simulink model "DataCenterCooling"  (R2025b)
settings: Solver=daessc  StartTime=0.0  StopTime=(env.nDays-1)*24*3600  MaxStep=60  RelTol=1e-3  AbsTol=1e-3
PreLoadFcn:
  | run("DataCenterCoolingExampleParams")
undefined symbols (not defined in the file or in its folder): cdu, Datacenter, ModelDatacenterLiquidCooling
libraries: fl_lib x101, SimscapeFluids_lib x27, nesl_utility x21, datacenter_lib x13, simulink_extras x2, slpidlib x1, buildingEnergy_lib x1
(part 1 of 3)
CloseFcn:
  | clear tout env cdu
Description:
  | Data Center Cooling
settings Model: Creator=The MathWorks, Inc.  LastModifiedBy=skota
settings SolverCC: AutoScaleAbsTol=off  MaxConsecutiveMinStep=500  AlgebraicLoopSolver=TrustRegion  MaxZcPerStep=1.0
settings DataIOCC: SaveOutput=off  DSMLogging=off  SaveTime=off  ReturnWorkspaceOutputs=off  SignalLoggingName=measurement_DataCenterCooling
settings OptimizationCC: ReuseModelBlockBuffer=off
settings DebuggingCC: UnconnectedInputMsg=warning  UnconnectedOutputMsg=warning  UnconnectedLineMsg=warning  SymbolicDimsDataTypeCodeGenerationDiagnostic=none
settings ModelReferenceCC: EnableRefExpFcnMdlSchedulingChecks=on
settings SFSimCC: CustomCodeUndefinedFunction=UseInterfaceOnly
settings RTWCC: GPUComputeCapability=3.5  DLArmComputeVersion=19.05
settings SimscapeCC: SimscapeLogType=all  SimscapeLogSimulationStatistics=on  SimscapeLogName=simlog_DataCenterCooling  SimscapeLogDataHistory=50000.0  SimscapeCompileComponentReuse=on

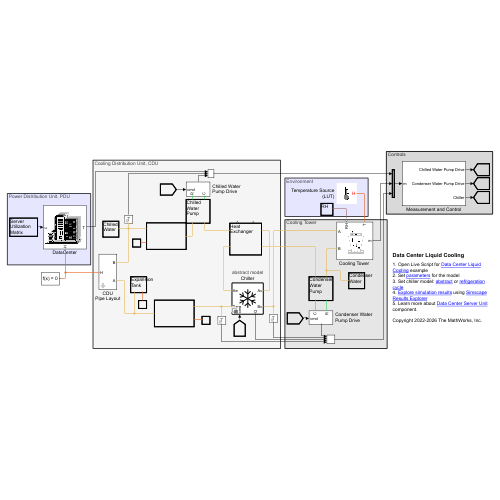
[thumbnail: Simulink's stored preview of the top-level diagram]
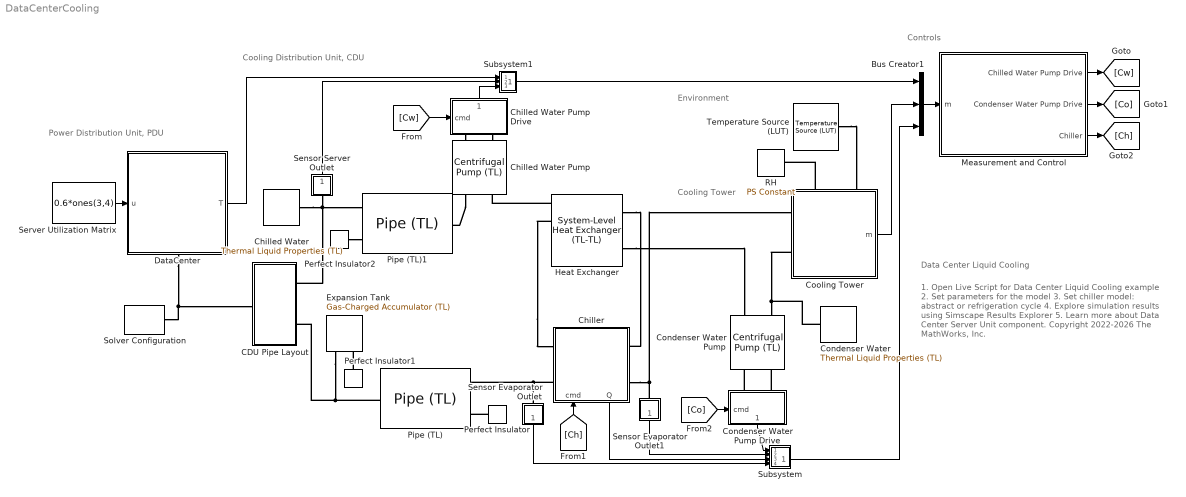
== system DataCenterCooling ==
  note: Controls
  note: Cooling Tower
  note: Environment
  note: Power Distribution Unit, PDU
  note: Cooling Distribution Unit, CDU
  note: Data Center Liquid Cooling
  note: 1. Open Live Script for Data Center Liquid Cooling example
      | 2. Set parameters for the model
      | 3. Set chiller model: abstract or refrigeration cycle
      | 4. Explore simulation results using Simscape Results Explorer
      | 5. Learn more about Data Center Server Unit component.
      |
      | Copyright 2022-2026 The MathWorks, Inc.
  Bus Creator1 : BusCreator  Inputs=3
  CDU Pipe Layout : Subsystem  mask{thRes=1e-5, distrDiameter=0.2, pipeDiameter=0.05, pipeLength=5}
      mask prompts: thRes "Thermal resistance (K/W)"; distrDiameter "Distributor pipe diameter (m)"; pipeDiameter "Cooling pipe diameter"; pipeLength "Pipe length (m)"
  Chilled Water : SimscapeFluids_lib/Thermal Liquid/Utilities/Thermal Liquid Properties (TL)  fluid_list=fluids.thermal_liquid.utilities.enum.thermal_liquid_fluid_list.ethylene_glycol  concentration_param_EG=fluids.thermal_liquid.utilities.enum.thermal_liquid_concentration.volume_fraction  concentration_param_PG=fluids.thermal_liquid.utilities.enum.thermal_liquid_concentration.volume_fraction  c_mass_SW=3.5e-3  c_mass_EG=0.1  c_mass_PG=0.1  c_mass_GL=0.1  c_vol_EG=0.3  c_vol_PG=0.1  beta_const_EG=2.1791 GPa  beta_const_PG=2.1791 GPa  beta_const_GL=2.1791 GPa  p_min_EG=0.01 MPa  p_min_PG=0.01 MPa  p_min_GL=0.01 MPa  p_max_EG=50 MPa  p_max_PG=50 MPa  p_max_GL=50 MPa  T_atm=293.15 K  p_atm=0.101325 MPa  properties_range_check=simscape.enum.assert.action.error  air_fraction=0  R_air=0.287 kJ/(K*kg)  air_dissolution_model=false  p_crit=3 MPa
  Chilled Water Pump : SimscapeFluids_lib/Thermal Liquid/Pumps & Motors/Centrifugal Pump (TL)  pump_parameterization=fluids.thermal_liquid.pumps_motors.enum.CentrifugalPumpParameterization.Nominal  capacity_ref_nominal=9600 lpm  head_ref_nominal=28 m  power_ref_nominal=60 kW  head_ref_max=40 m  capacity_ref_max=15000 lpm  omega_ref_analytic=2400 rpm  flow_rate_1D_TLU=[16.67, 30, 40, 53.33, 66.67, 83.33] lpm  head_1D_TLU=[50, 47.5, 45, 40, 35, 25] m  power_1D_TLU=[.6, .75, .85, .93, .98, .99] kW  omega_ref_1D=3500 rpm  rho_ref_1D=998.21 kg/m^3  omega_threshold_factor=1e-2  flow_rate_2D_TLU=[16.67, 23.33, 30, 40, 53.33, 60] lpm  omega_2D_TLU=[2450, 2800, 3150, 3500] rpm  head_2D_TLU=[25, 32.7, 42.5, 50; 24, 31.7, 41, 49; 22.7, 30.5, 39, 47.5; 20, 28, 36, 45; 15.7, 24, 32, 40; 12.5, 21, 29.5, 37.5] m  power_2D_TLU=[.28, .38, .5, .6; .31, .41, .55, .68; .33, .44, .6, .75; .36, .48, .65, .83; .38, .53, .72, .93; .39, .55, .75, .97] kW  rho_ref_2D=998.21 kg/m^3  diameter_ratio=1  mech_orientation=fluids.thermal_liquid.pumps_motors.enum.CentrifugalPumpMechOrientation.Positive  area=cdu.port_area m^2  operation_check=simscape.enum.assert.action.none
  Chilled Water Pump Drive : Subsystem
      settings: PortSchema="{\"entries\":[{\"content\":{\"sides\":[{\"content\":{},\"type\":\"ConnectorPlacement.EquallySpacedRectSide\",\"uuid\":\"edaea338-c02b-45e4-bb82-2d3d355c0ecb\"},{\"content\":{\"connectorIds\":[\"In1\"],\"side\":\"RIGHT\"},\"type\":\"ConnectorPlacement.EquallySpacedRectSide\",\"uuid\":\"dbf9c5c1-eafd-40d4-aa46-26e8ea9aa192\"},{\"content\":{\"connectorIds\":[\"LConn1\",\"LConn2\"],\"side\":\"TOP\"},\"type\":\"ConnectorPlacement.EquallySpacedRectSide\",\"uuid\":\"608efdba-9ff5-4da4-84d8-d12421fbb1b5\"},{\"content\":{\"connectorIds\":[\"Out1\"],\"side\":\"BOTTOM\"},\"type\":\"ConnectorPlacement.EquallySpacedRectSide\",\"uuid\":\"72b6a2af-375d-4ab8-a644-645304dfa2ef\"}]},\"type\":\"ConnectorPlacement.EquallySpacedConnector\",\"uuid\":\"d68ea5d9-0a41-4434-9ea5-6f17886b9eb3\"}],\"packageUris\":[\"http://schema.mathworks.com/mf0/Connector/R2020b\"],\"version\":\"1.0\"}"
  Chiller : Subsystem  Variant=on  VariantControlMode=label  LabelModeActiveChoice=abstract model
      settings: AttributesFormatString=%<LabelModeActiveChoice>  PortSchema="{\"entries\":[{\"content\":{\"sides\":[{\"content\":{\"connectorIds\":[\"LConn1\",\"LConn2\"]},\"type\":\"ConnectorPlacement.EquallySpacedRectSide\",\"uuid\":\"5ef38cea-bb7b-401a-87d4-4f5e5e2c1e9f\"},{\"content\":{\"connectorIds\":[\"RConn1\",\"RConn2\"],\"side\":\"RIGHT\"},\"type\":\"ConnectorPlacement.EquallySpacedRectSide\",\"uuid\":\"7c200196-8d5a-4dde-899e-2352968f9ffc\"},{\"content\":{\"side\":\"TOP\"},\"type\":\"ConnectorPlacement.EquallySpacedRectSide\",\"uuid\":\"5e8cb91d-7f29-4d1c-a98e-548e0eb69733\"},{\"content\":{\"connectorIds\":[\"In1\",\"Out1\"],\"side\":\"BOTTOM\"},\"type\":\"ConnectorPlacement.EquallySpacedRectSide\",\"uuid\":\"d3cfe7a1-f14c-45f3-9f19-8fd891085d29\"}]},\"type\":\"ConnectorPlacement.EquallySpacedConnector\",\"uuid\":\"25b6c22e-1b50-48b1-b598-85423fadd037\"}],\"packageUris\":[\"http://schema.mathworks.com/mf0/Connector/R2020b\"],\"version\":\"1.0\"}"
      mask Display:
      | plot([-100 100 100 -100 -100], [-100 -100 100 100 -100])
      | 
      | % Width and height scale factors
      | w = 60;
      | h = 60;
      | 
      | % Coordinates [x; y]
      | trunk = [0 0; -1 1];
      | tip1 = [-0.3 0 0.3; 0.8 0.5 0.8];
      | tip2 = [-0.3 0 0.3; -0.8 -0.5 -0.8];
      | 
      | % Vertical line
      | plot(w*trunk(1,:), h*trunk(2,:))
      | plot(w*tip1(1,:), h*tip1(2,:))
      | plot(w*tip2(1,:), h*tip2(2,:))
      | 
      | % Rotate 60 deg
      | theta = 60;
      | rot = [cosd(theta) -sind(theta); sind(theta) cosd(theta)];
      | trunk_rot = rot*trunk;
      | tip1_rot = rot*tip1;
      | tip2_rot = rot*tip2;
      | plot(w*trunk_rot(1,:), h*trunk_rot(2,:))
      | plot(w*tip1_rot(1,:), h*tip1_rot(2,:))
      | plot(w*tip2_rot(1,:), h*tip2_rot(2,:))
      | 
      | % Rotate 120 deg
      | theta = 120;
      | rot = [cosd(theta) -sind(theta); sind(theta) cosd(theta)];
      | trunk_rot = rot*trunk;
      | tip1_rot = rot*tip1;
      | tip2_rot = rot*tip2;
      | plot(w*trunk_rot(1,:), h*trunk_rot(2,:))
      | plot(w*tip1_rot(1,:), h*tip1_rot(2,:))
      | plot(w*tip2_rot(1,:), h*tip2_rot(2,:))
  Condenser Water : SimscapeFluids_lib/Thermal Liquid/Utilities/Thermal Liquid Properties (TL)  fluid_list=fluids.thermal_liquid.utilities.enum.thermal_liquid_fluid_list.water  concentration_param_EG=fluids.thermal_liquid.utilities.enum.thermal_liquid_concentration.volume_fraction  concentration_param_PG=fluids.thermal_liquid.utilities.enum.thermal_liquid_concentration.volume_fraction  c_mass_SW=3.5e-3  c_mass_EG=0.1  c_mass_PG=0.1  c_mass_GL=0.1  c_vol_EG=0.1  c_vol_PG=0.1  beta_const_EG=2.1791 GPa  beta_const_PG=2.1791 GPa  beta_const_GL=2.1791 GPa  p_min_EG=0.01 MPa  p_min_PG=0.01 MPa  p_min_GL=0.01 MPa  p_max_EG=50 MPa  p_max_PG=50 MPa  p_max_GL=50 MPa  T_atm=293.15 K  p_atm=0.101325 MPa  properties_range_check=simscape.enum.assert.action.error  air_fraction=0  R_air=0.287 kJ/(K*kg)  air_dissolution_model=false  p_crit=3 MPa
  Condenser Water Pump : SimscapeFluids_lib/Thermal Liquid/Pumps & Motors/Centrifugal Pump (TL)  pump_parameterization=fluids.thermal_liquid.pumps_motors.enum.CentrifugalPumpParameterization.Nominal  capacity_ref_nominal=15000 lpm  head_ref_nominal=33 m  power_ref_nominal=100 kW  head_ref_max=48 m  capacity_ref_max=24000 lpm  omega_ref_analytic=2400 rpm  flow_rate_1D_TLU=[16.67, 30, 40, 53.33, 66.67, 83.33] lpm  head_1D_TLU=[50, 47.5, 45, 40, 35, 25] m  power_1D_TLU=[.6, .75, .85, .93, .98, .99] kW  omega_ref_1D=3500 rpm  rho_ref_1D=998.21 kg/m^3  omega_threshold_factor=1e-2  flow_rate_2D_TLU=[16.67, 23.33, 30, 40, 53.33, 60] lpm  omega_2D_TLU=[2450, 2800, 3150, 3500] rpm  head_2D_TLU=[25, 32.7, 42.5, 50; 24, 31.7, 41, 49; 22.7, 30.5, 39, 47.5; 20, 28, 36, 45; 15.7, 24, 32, 40; 12.5, 21, 29.5, 37.5] m  power_2D_TLU=[.28, .38, .5, .6; .31, .41, .55, .68; .33, .44, .6, .75; .36, .48, .65, .83; .38, .53, .72, .93; .39, .55, .75, .97] kW  rho_ref_2D=998.21 kg/m^3  diameter_ratio=1  mech_orientation=fluids.thermal_liquid.pumps_motors.enum.CentrifugalPumpMechOrientation.Positive  area=cdu.port_area m^2  operation_check=simscape.enum.assert.action.none
  Condenser Water Pump Drive : Subsystem
      settings: PortSchema="{\"entries\":[{\"content\":{\"sides\":[{\"content\":{\"connectorIds\":[\"In1\"]},\"type\":\"ConnectorPlacement.EquallySpacedRectSide\",\"uuid\":\"edaea338-c02b-45e4-bb82-2d3d355c0ecb\"},{\"content\":{\"side\":\"RIGHT\"},\"type\":\"ConnectorPlacement.EquallySpacedRectSide\",\"uuid\":\"dbf9c5c1-eafd-40d4-aa46-26e8ea9aa192\"},{\"content\":{\"connectorIds\":[\"LConn1\",\"LConn2\"],\"side\":\"TOP\"},\"type\":\"ConnectorPlacement.EquallySpacedRectSide\",\"uuid\":\"608efdba-9ff5-4da4-84d8-d12421fbb1b5\"},{\"content\":{\"connectorIds\":[\"Out1\"],\"side\":\"BOTTOM\"},\"type\":\"ConnectorPlacement.EquallySpacedRectSide\",\"uuid\":\"608ab80a-f5e8-4836-b78e-f2f30ba8946b\"}]},\"type\":\"ConnectorPlacement.EquallySpacedConnector\",\"uuid\":\"d68ea5d9-0a41-4434-9ea5-6f17886b9eb3\"}],\"packageUris\":[\"http://schema.mathworks.com/mf0/Connector/R2020b\"],\"version\":\"1.0\"}"
  "Cooling Tower " : Subsystem
      settings: PortSchema="{\"entries\":[{\"content\":{\"sides\":[{\"content\":{\"connectorIds\":[\"LConn1\",\"LConn2\"]},\"type\":\"ConnectorPlacement.EquallySpacedRectSide\",\"uuid\":\"fb95f023-248b-4fd8-b2e8-d9442f9ed266\"},{\"content\":{\"connectorIds\":[\"Out1\"],\"side\":\"RIGHT\"},\"type\":\"ConnectorPlacement.EquallySpacedRectSide\",\"uuid\":\"34018b48-7083-4d8d-9b59-330dd3458507\"},{\"content\":{\"connectorIds\":[\"LConn3\",\"LConn4\"],\"side\":\"TOP\"},\"type\":\"ConnectorPlacement.EquallySpacedRectSide\",\"uuid\":\"5b7035e5-549d-4a54-bb0d-bc476d1d6775\"}]},\"type\":\"ConnectorPlacement.EquallySpacedConnector\",\"uuid\":\"c33b1996-e402-4893-a457-f5cd841aa14c\"}],\"packageUris\":[\"http://schema.mathworks.com/mf0/Connector/R2020b\"],\"version\":\"1.0\"}"
      mask Display: image('coolingTowerIcon.png');
  DataCenter : Subsystem
      settings: PortSchema="{\"entries\":[{\"content\":{\"sides\":[{\"content\":{\"connectorIds\":[\"In1\"]},\"type\":\"ConnectorPlacement.EquallySpacedRectSide\",\"uuid\":\"0d94ea3d-d897-456d-b7bd-42d620e46e28\"},{\"content\":{\"connectorIds\":[\"Out1\"],\"side\":\"RIGHT\"},\"type\":\"ConnectorPlacement.EquallySpacedRectSide\",\"uuid\":\"b45d02ac-efb1-4fbd-bb62-56ba599fe73d\"},{\"content\":{\"side\":\"TOP\"},\"type\":\"ConnectorPlacement.EquallySpacedRectSide\",\"uuid\":\"5c5ba700-ead5-48ef-be98-ffdeec5238e7\"},{\"content\":{\"connectorIds\":[\"RConn1\"],\"side\":\"BOTTOM\"},\"type\":\"ConnectorPlacement.EquallySpacedRectSide\",\"uuid\":\"4fcdfdd2-a15c-4a40-81f5-7d3c5a9fd94e\"}]},\"type\":\"ConnectorPlacement.EquallySpacedConnector\",\"uuid\":\"41bff309-caa4-4da4-abd9-c4b3acd5f02a\"}],\"packageUris\":[\"http://schema.mathworks.com/mf0/Connector/R2020b\"],\"version\":\"1.0\"}"
      mask Display: image('datacenter.png');
  Expansion Tank : SimscapeFluids_lib/Thermal Liquid/Tanks & Accumulators/Gas-Charged Accumulator (TL)  capacity=1 m^3  dead_volume=1e-3 m^3  p_precharge_gauge=0.28 MPa  k_sh=1.4  area=cdu.port_area m^2  stiff_coeff=1e4 MPa/m^3  damping_coeff=1e4 MPa*s/m^6  liquid_volume_specify=on  liquid_volume_priority=None  liquid_volume=5e-3 m^3  liquid_volume_nominal_specify=off  liquid_volume_nominal_value=1  liquid_volume_nominal_unit=m^3  liquid_mass_specify=off  liquid_mass_priority=None  liquid_mass=5 kg  liquid_mass_nominal_specify=off  liquid_mass_nominal_value=1  liquid_mass_nominal_unit=kg  p_I_specify=on  p_I_priority=High  p_I=0.4 MPa  p_I_nominal_specify=off  p_I_nominal_value=1  p_I_nominal_unit=MPa  T_I_specify=on  T_I_priority=High  T_I=18 degC  T_I_nominal_specify=off  T_I_nominal_value=1  T_I_nominal_unit=K
  Heat Exchanger : SimscapeFluids_lib/Heat Exchangers/Thermal Liquid/System-Level Heat Exchanger (TL-TL)  flow_arrangement=fluids.heat_exchangers.enum.SystemLevelFlowArrangementTLTL.Counter  wall_thermal_mass=false  mass_wall=1 kg  cp_wall=490 J/(K*kg)  nominal_init_wall=true  T_wall_init=293.15 K  area_A1=cdu.port_area m^2  area_B1=cdu.port_area m^2  area_A2=cdu.port_area m^2  area_B2=cdu.port_area m^2  operating_condition_TL1=fluids.heat_exchangers.enum.SystemLevelOperatingConditionTLTL.Cooling  mdot_nominal_TL1=160 kg/s  delta_p_nominal_TL1=0.1 MPa  p_in_nominal_TL1=0.6 MPa  T_in_nominal_TL1=28 degC  capacity_spec_TL1=fluids.heat_exchangers.enum.SystemLevelCapacitySpec.HeatTransfer  Q_nominal=3000 kW  T_out_nominal_TL1=323.15 K  volume_TL1=2 m^3  nominal_init_TL1=true  p_init_TL1=0.101325 MPa  T_init_TL1=293.15 K  mdot_nominal_TL2=250 kg/s  delta_p_nominal_TL2=0.2 MPa  p_in_nominal_TL2=0.4 MPa  T_in_nominal_TL2=22 degC  volume_TL2=2 m^3  nominal_init_TL2=true  p_init_TL2=0.101325 MPa  T_init_TL2=293.15 K  a_TL1=0.023  b_TL1=0.8  c_TL1=0.33  a_TL2=0.023  b_TL2=0.8  c_TL2=0.33
  Measurement and Control : Subsystem
  Perfect Insulator : fl_lib/Thermal/Thermal Elements/Perfect Insulator  T_specify=off  T_priority=None  T=293.15 K  T_nominal_specify=off  T_nominal_value=1  T_nominal_unit=K
  Perfect Insulator1 : fl_lib/Thermal/Thermal Elements/Perfect Insulator  T_specify=off  T_priority=None  T=293.15 K  T_nominal_specify=off  T_nominal_value=1  T_nominal_unit=K
  Perfect Insulator2 : fl_lib/Thermal/Thermal Elements/Perfect Insulator  T_specify=off  T_priority=None  T=293.15 K  T_nominal_specify=off  T_nominal_value=1  T_nominal_unit=K
  Pipe (TL) : SimscapeFluids_lib/Thermal Liquid/Pipes & Fittings/Pipe (TL)  dynamic_compressibility=true  inertia=false  num_segments=1  pipe_length=10 m  cross_section_geometry=fluids.thermal_liquid.pipes_fittings.enum.CrossSectionGeometry.Custom  pipe_diameter=0.1 m  pipe_inner_diameter=0.05 m  pipe_outer_diameter=0.1 m  pipe_width=0.1 m  pipe_height=0.1 m  pipe_major_axis=0.1 m  pipe_minor_axis=0.05 m  pipe_side=0.1 m  pipe_angle=30 deg  area=pi*0.05^2/4 * 30 m^2  Dh=0.05 m  elevation_spec=foundation.enum.constant_variable.constant  elevation_gain=0 m  gravity_spec=foundation.enum.constant_variable.constant  g=9.81 m/s^2  pressure_loss_spec=fluids.thermal_liquid.pipes_fittings.enum.PressureLossSpec.Haaland  local_pressure_loss_spec=fluids.thermal_liquid.pipes_fittings.enum.LocalLossSpec.LossCoefficient  length_add=1 m  loss_coefficient=1  roughness_spec=fluids.thermal_liquid.pipes_fittings.enum.RoughnessSpec.Custom  roughness=15e-6 m  Re_friction_TLU=[400, 1000, 1500, 3000, 4000, 6000, 10000, 20000, 40000, 60000, 100000, 100000000]  friction_factor_TLU=[.264, .112, .071, .0417, .0387, .0268, .025, .0232, .0226, .022, .0214, .0214]  Re_lam=2000  Re_tur=4000  shape_factor=64  mdot_nominal=[.1, 1] kg/s  p_diff_nominal=[.001, .01] MPa  mdot_threshold=1e-6 kg/s  wall_spec=fluids.thermal_liquid.pipes_fittings.enum.wall_spec.rigid  vol_expansion_spec=fluids.thermal_liquid.pipes_fittings.enum.VolumeExpansionSpec.Diameter  area_pressure_gain=1e-6 m^2/MPa  static_pressure_TLU=[.1, 1] MPa  area_pressure_gain_TLU=[1e-05, 1.1e-05] m^2  material_behavior_spec=fluids.thermal_liquid.pipes_fittings.enum.PipeMaterialBehavior.Linear  diameter_pressure_gain=1e-6 m/MPa  wall_thickness=0.05 m  elastic_modulus=69 GPa  stress_TLU=[276, 310] MPa  strain_TLU=[.004, .02]  stress_assert_action=simscape.enum.assert.action.none  stress_max=400 MPa  poisson_ratio=0.33  wall_time_constant=0.01 s  thermal_expansion=false  alpha_L_wall=24 um/(deltaK*m)  thermal_expansion_Tref=293.15 K  heat_transfer_spec=fluids.thermal_liquid.pipes_fittings.enum.HeatTransferSpec.Gnielinski  mdot_nominal_heat=[.1, 1] kg/s  T_in_nominal=[293.15, 293.15] K  T_out_nominal=[300, 300] K  p_in_nominal_heat=[.101325, .101325] MPa  T_wall_nominal=[303.15, 303.15] K  a_coeff=0.023  b_Re_power=0.8  c_Pr_power=0.4  Nu_lam=3.66  Re_Colburn_TLU=[100, 150, 1000]  Colburn_factor_TLU=[.019, .013, .002]  Re_Nu_TLU=[100, 150, 1000]  Pr_Nu_TLU=[1, 10]  Nu_TLU=[3.72, 4.21; 3.75, 4.44; 4.21, 7.15]  p0_vec=0.4 MPa  T0_vec=18 degC  mdot0=0.1 kg/s  p_nominal=0.101325 MPa  T_nominal=293.15 K
  Pipe (TL)1 : SimscapeFluids_lib/Thermal Liquid/Pipes & Fittings/Pipe (TL)  dynamic_compressibility=true  inertia=false  num_segments=1  pipe_length=10 m  cross_section_geometry=fluids.thermal_liquid.pipes_fittings.enum.CrossSectionGeometry.Custom  pipe_diameter=0.1 m  pipe_inner_diameter=0.05 m  pipe_outer_diameter=0.1 m  pipe_width=0.1 m  pipe_height=0.1 m  pipe_major_axis=0.1 m  pipe_minor_axis=0.05 m  pipe_side=0.1 m  pipe_angle=30 deg  area=pi*0.05^2/4 * 30 m^2  Dh=0.05 m  elevation_spec=foundation.enum.constant_variable.constant  elevation_gain=0 m  gravity_spec=foundation.enum.constant_variable.constant  g=9.81 m/s^2  pressure_loss_spec=fluids.thermal_liquid.pipes_fittings.enum.PressureLossSpec.Haaland  local_pressure_loss_spec=fluids.thermal_liquid.pipes_fittings.enum.LocalLossSpec.LossCoefficient  length_add=1 m  loss_coefficient=1  roughness_spec=fluids.thermal_liquid.pipes_fittings.enum.RoughnessSpec.Custom  roughness=15e-6 m  Re_friction_TLU=[400, 1000, 1500, 3000, 4000, 6000, 10000, 20000, 40000, 60000, 100000, 100000000]  friction_factor_TLU=[.264, .112, .071, .0417, .0387, .0268, .025, .0232, .0226, .022, .0214, .0214]  Re_lam=2000  Re_tur=4000  shape_factor=64  mdot_nominal=[.1, 1] kg/s  p_diff_nominal=[.001, .01] MPa  mdot_threshold=1e-6 kg/s  wall_spec=fluids.thermal_liquid.pipes_fittings.enum.wall_spec.rigid  vol_expansion_spec=fluids.thermal_liquid.pipes_fittings.enum.VolumeExpansionSpec.Diameter  area_pressure_gain=1e-6 m^2/MPa  static_pressure_TLU=[.1, 1] MPa  area_pressure_gain_TLU=[1e-05, 1.1e-05] m^2  material_behavior_spec=fluids.thermal_liquid.pipes_fittings.enum.PipeMaterialBehavior.Linear  diameter_pressure_gain=1e-6 m/MPa  wall_thickness=0.05 m  elastic_modulus=69 GPa  stress_TLU=[276, 310] MPa  strain_TLU=[.004, .02]  stress_assert_action=simscape.enum.assert.action.none  stress_max=400 MPa  poisson_ratio=0.33  wall_time_constant=0.01 s  thermal_expansion=false  alpha_L_wall=24 um/(deltaK*m)  thermal_expansion_Tref=293.15 K  heat_transfer_spec=fluids.thermal_liquid.pipes_fittings.enum.HeatTransferSpec.Gnielinski  mdot_nominal_heat=[.1, 1] kg/s  T_in_nominal=[293.15, 293.15] K  T_out_nominal=[300, 300] K  p_in_nominal_heat=[.101325, .101325] MPa  T_wall_nominal=[303.15, 303.15] K  a_coeff=0.023  b_Re_power=0.8  c_Pr_power=0.4  Nu_lam=3.66  Re_Colburn_TLU=[100, 150, 1000]  Colburn_factor_TLU=[.019, .013, .002]  Re_Nu_TLU=[100, 150, 1000]  Pr_Nu_TLU=[1, 10]  Nu_TLU=[3.72, 4.21; 3.75, 4.44; 4.21, 7.15]  p0_vec=0.4 MPa  T0_vec=28 degC  mdot0=0.1 kg/s  p_nominal=0.101325 MPa  T_nominal=293.15 K
  RH : fl_lib/Physical Signals/Sources/PS Constant  constant=0.6
  Sensor Evaporator Outlet : Subsystem
      mask Display: disp('T')
  Sensor Evaporator Outlet1 : Subsystem
      mask Display: disp('T')
  Sensor Server Outlet : Subsystem
      mask Display: disp('T')
  Server Utilization Matrix : Constant  Value=0.6*ones(3,4)
  Solver Configuration : nesl_utility/Solver Configuration  PhysicalDomain=network_engine_domain  SubClassName=solver  LeftPortType=input  RightPortType=generic  Tones=[]  Harmonics=[]  SimulateNoise=off  Profile=off  UseLocalSampling=off  EnableSwitchedLinearOptims=on  FrequencyDomain=off  UseCCode=off  RelTol=0.001  AbsTol=0.001  MinStep=1e-09  ToWorkspace=off  RevertToSquareIcSolve=off  NumHomotopyIterations=100  PhasorMode=off  PhasorModeNumHarmonics=1  ConsistencySolver=NEWTON_XTOL_AFTER_FTOL  CanonicalOrdering=UNORDERED  OptimizeIntermediates=UNOPTIMIZED  IndexReductionMethod=None  DoDC=off  ResidualTolerance=1e-09  ConsistencyTolSource=GLOBAL  ConsistencyAbsTol=0.001  ConsistencyRelTol=0.001  ConsistencyTolFactor=0.001  UseLocalSolver=off  LocalSolverChoice=NE_BACKWARD_EULER_ADVANCER  ResolveIndetEquations=on  FunctionEvalNumThread=1  LocalSolverSampleTime=0.001  DoFixedCost=off  MaxNonlinIter=3  MaxModeIter=2  ComputeImpulses=off  ImpulseIterations=2  LinearAlgebra=auto  LinearAlgebraNumThread=0  EquationFormulation=NE_TIME_EF  DelaysMemoryBudget=1024  AutomaticFiltering=on  FilteringTimeConstant=0.001  PartitionStorageMethod=AS_NEEDED  PartitionMemoryBudget=1024  PartitionMethod=ROBUST  MultibodyUseLocalSolver=off  MultibodyLocalSolverChoice=ODE1  MultibodyLocalSolverSampleTime=0.001
  Subsystem : Subsystem
  Subsystem1 : Subsystem
  Temperature Source (LUT) : buildingEnergy_lib/Temperature Source (LUT)  latitude=env.latitude  longitude=env.longitude  localTime=env.refLongitude  dayLightS=0  startYear=env.startYear  startMonth=env.startMonth  startDay=env.startDate  startHr=env.startHour  numDaysData=env.nDays  interp_method=simscape.enum.interpolation.linear  extrap_method=simscape.enum.extrapolation.error  avgDayTvec=env.dayTvec K  pcDayTvar=5  avgNightTvec=env.nightTvec K  pcNightTvar=5
  wires:
  Condenser Water Pump Drive/1(" ") -> Subsystem/1("    ")
  Chiller/1(Q) -> Subsystem/3("   ")
  Sensor Evaporator Outlet1/1(Tcond) -> Subsystem/2("  ")
  Sensor Evaporator Outlet/1(Tevap) -> Subsystem/4(" ")
  Chilled Water Pump Drive/1(" ") -> Subsystem1/3("   ")
  Sensor Server Outlet/1(Ts,fluid) -> Subsystem1/2("  ")
  Measurement and Control/1(Chilled Water Pump Drive) -> [Cw]
  Measurement and Control/2(Condenser Water Pump Drive) -> [Co]
  Measurement and Control/3(Chiller) -> [Ch]
  [Cw] -> Chilled Water Pump Drive/1(cmd)
  [Ch] -> Chiller/1(cmd)
  [Co] -> Condenser Water Pump Drive/1(cmd)
  "Cooling Tower "/1(m) -> Bus Creator1/2
  Subsystem1/1("    ") -> Bus Creator1/1
  Subsystem/1("     ") -> Bus Creator1/3
  Bus Creator1/1 -> Measurement and Control/1(m)
  Server Utilization Matrix/1 -> DataCenter/1(u)
  DataCenter/1(T) -> Subsystem1/1(" ")
  connections:
  Perfect Insulator/LConn1 -- Pipe (TL)/LConn2
  Perfect Insulator2/LConn1 -- Pipe (TL)1/LConn2
  Perfect Insulator1/LConn1 -- Expansion Tank/RConn2
  Chilled Water Pump/LConn1 -- Pipe (TL)1/RConn1
  Heat Exchanger/LConn2 -- Chiller/LConn1
  Chiller/LConn2 -- Sensor Evaporator Outlet/LConn1 -- Pipe (TL)/LConn1
  Chilled Water Pump Drive/LConn2 -- Chilled Water Pump/RConn1
  Chilled Water Pump Drive/LConn1 -- Chilled Water Pump/RConn2
  Heat Exchanger/RConn1 -- Chiller/RConn1
  Heat Exchanger/RConn2 -- Condenser Water Pump/LConn2
  Chiller/RConn2 -- Sensor Evaporator Outlet1/LConn1 -- "Cooling Tower "/LConn1
  "Cooling Tower "/LConn2 -- Condenser Water/RConn1 -- Condenser Water Pump/LConn1
  Condenser Water Pump Drive/LConn1 -- Condenser Water Pump/RConn2
  Condenser Water Pump Drive/LConn2 -- Condenser Water Pump/RConn1
  Heat Exchanger/LConn1 -- Chilled Water Pump/LConn2
  "Cooling Tower "/LConn3 -- RH/RConn1
  Chilled Water/RConn1 -- Pipe (TL)1/LConn1 -- CDU Pipe Layout/RConn1 -- Sensor Server Outlet/LConn1
  Pipe (TL)/RConn1 -- CDU Pipe Layout/RConn2 -- Expansion Tank/RConn1
  Temperature Source (LUT)/RConn1 -- "Cooling Tower "/LConn4
  DataCenter/RConn1 -- CDU Pipe Layout/LConn1 -- Solver Configuration/RConn1

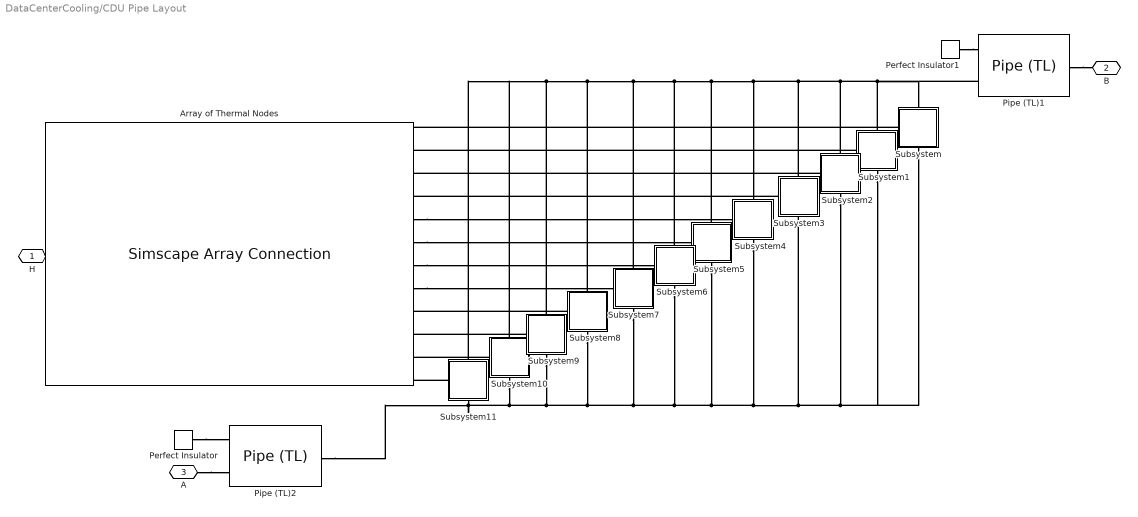
== system DataCenterCooling/CDU Pipe Layout ==
  Array of Thermal Nodes : SimscapeArrayConnection  Domain=foundation.thermal.thermal  ConcatenateDimension=1  NumScalarElements=12
  Perfect Insulator : fl_lib/Thermal/Thermal Elements/Perfect Insulator  T_specify=off  T_priority=None  T=293.15 K  T_nominal_specify=off  T_nominal_value=1  T_nominal_unit=K
  Perfect Insulator1 : fl_lib/Thermal/Thermal Elements/Perfect Insulator  T_specify=off  T_priority=None  T=293.15 K  T_nominal_specify=off  T_nominal_value=1  T_nominal_unit=K
  Pipe (TL)1 : SimscapeFluids_lib/Thermal Liquid/Pipes & Fittings/Pipe (TL)  dynamic_compressibility=true  inertia=false  num_segments=1  pipe_length=pipeLength m  cross_section_geometry=fluids.thermal_liquid.pipes_fittings.enum.CrossSectionGeometry.Custom  pipe_diameter=0.1 m  pipe_inner_diameter=0.05 m  pipe_outer_diameter=0.1 m  pipe_width=0.1 m  pipe_height=0.1 m  pipe_major_axis=0.1 m  pipe_minor_axis=0.05 m  pipe_side=0.1 m  pipe_angle=30 deg  area=pi*distrDiameter^2/4 m^2  Dh=distrDiameter m  elevation_spec=foundation.enum.constant_variable.constant  elevation_gain=0 m  gravity_spec=foundation.enum.constant_variable.constant  g=9.81 m/s^2  pressure_loss_spec=fluids.thermal_liquid.pipes_fittings.enum.PressureLossSpec.Haaland  local_pressure_loss_spec=fluids.thermal_liquid.pipes_fittings.enum.LocalLossSpec.LossCoefficient  length_add=1 m  loss_coefficient=1  roughness_spec=fluids.thermal_liquid.pipes_fittings.enum.RoughnessSpec.Custom  roughness=15e-6 m  Re_friction_TLU=[400, 1000, 1500, 3000, 4000, 6000, 10000, 20000, 40000, 60000, 100000, 100000000]  friction_factor_TLU=[.264, .112, .071, .0417, .0387, .0268, .025, .0232, .0226, .022, .0214, .0214]  Re_lam=2000  Re_tur=4000  shape_factor=64  mdot_nominal=[.1, 1] kg/s  p_diff_nominal=[.001, .01] MPa  mdot_threshold=1e-6 kg/s  wall_spec=fluids.thermal_liquid.pipes_fittings.enum.wall_spec.rigid  vol_expansion_spec=fluids.thermal_liquid.pipes_fittings.enum.VolumeExpansionSpec.Diameter  area_pressure_gain=1e-6 m^2/MPa  static_pressure_TLU=[.1, 1] MPa  area_pressure_gain_TLU=[1e-05, 1.1e-05] m^2  material_behavior_spec=fluids.thermal_liquid.pipes_fittings.enum.PipeMaterialBehavior.Linear  diameter_pressure_gain=1e-6 m/MPa  wall_thickness=0.05 m  elastic_modulus=69 GPa  stress_TLU=[276, 310] MPa  strain_TLU=[.004, .02]  stress_assert_action=simscape.enum.assert.action.none  stress_max=400 MPa  poisson_ratio=0.33  wall_time_constant=0.01 s  thermal_expansion=false  alpha_L_wall=24 um/(deltaK*m)  thermal_expansion_Tref=293.15 K  heat_transfer_spec=fluids.thermal_liquid.pipes_fittings.enum.HeatTransferSpec.Gnielinski  mdot_nominal_heat=[.1, 1] kg/s  T_in_nominal=[293.15, 293.15] K  T_out_nominal=[300, 300] K  p_in_nominal_heat=[.101325, .101325] MPa  T_wall_nominal=[303.15, 303.15] K  a_coeff=0.023  b_Re_power=0.8  c_Pr_power=0.4  Nu_lam=3.66  Re_Colburn_TLU=[100, 150, 1000]  Colburn_factor_TLU=[.019, .013, .002]  Re_Nu_TLU=[100, 150, 1000]  Pr_Nu_TLU=[1, 10]  Nu_TLU=[3.72, 4.21; 3.75, 4.44; 4.21, 7.15]  p0_vec=0.4 MPa  T0_vec=28 degC  mdot0=0.1 kg/s  p_nominal=0.101325 MPa  T_nominal=293.15 K
  Pipe (TL)2 : SimscapeFluids_lib/Thermal Liquid/Pipes & Fittings/Pipe (TL)  dynamic_compressibility=true  inertia=false  num_segments=1  pipe_length=pipeLength m  cross_section_geometry=fluids.thermal_liquid.pipes_fittings.enum.CrossSectionGeometry.Custom  pipe_diameter=0.1 m  pipe_inner_diameter=0.05 m  pipe_outer_diameter=0.1 m  pipe_width=0.1 m  pipe_height=0.1 m  pipe_major_axis=0.1 m  pipe_minor_axis=0.05 m  pipe_side=0.1 m  pipe_angle=30 deg  area=pi*distrDiameter^2/4 m^2  Dh=distrDiameter m  elevation_spec=foundation.enum.constant_variable.constant  elevation_gain=0 m  gravity_spec=foundation.enum.constant_variable.constant  g=9.81 m/s^2  pressure_loss_spec=fluids.thermal_liquid.pipes_fittings.enum.PressureLossSpec.Haaland  local_pressure_loss_spec=fluids.thermal_liquid.pipes_fittings.enum.LocalLossSpec.LossCoefficient  length_add=1 m  loss_coefficient=1  roughness_spec=fluids.thermal_liquid.pipes_fittings.enum.RoughnessSpec.Custom  roughness=15e-6 m  Re_friction_TLU=[400, 1000, 1500, 3000, 4000, 6000, 10000, 20000, 40000, 60000, 100000, 100000000]  friction_factor_TLU=[.264, .112, .071, .0417, .0387, .0268, .025, .0232, .0226, .022, .0214, .0214]  Re_lam=2000  Re_tur=4000  shape_factor=64  mdot_nominal=[.1, 1] kg/s  p_diff_nominal=[.001, .01] MPa  mdot_threshold=1e-6 kg/s  wall_spec=fluids.thermal_liquid.pipes_fittings.enum.wall_spec.rigid  vol_expansion_spec=fluids.thermal_liquid.pipes_fittings.enum.VolumeExpansionSpec.Diameter  area_pressure_gain=1e-6 m^2/MPa  static_pressure_TLU=[.1, 1] MPa  area_pressure_gain_TLU=[1e-05, 1.1e-05] m^2  material_behavior_spec=fluids.thermal_liquid.pipes_fittings.enum.PipeMaterialBehavior.Linear  diameter_pressure_gain=1e-6 m/MPa  wall_thickness=0.05 m  elastic_modulus=69 GPa  stress_TLU=[276, 310] MPa  strain_TLU=[.004, .02]  stress_assert_action=simscape.enum.assert.action.none  stress_max=400 MPa  poisson_ratio=0.33  wall_time_constant=0.01 s  thermal_expansion=false  alpha_L_wall=24 um/(deltaK*m)  thermal_expansion_Tref=293.15 K  heat_transfer_spec=fluids.thermal_liquid.pipes_fittings.enum.HeatTransferSpec.Gnielinski  mdot_nominal_heat=[.1, 1] kg/s  T_in_nominal=[293.15, 293.15] K  T_out_nominal=[300, 300] K  p_in_nominal_heat=[.101325, .101325] MPa  T_wall_nominal=[303.15, 303.15] K  a_coeff=0.023  b_Re_power=0.8  c_Pr_power=0.4  Nu_lam=3.66  Re_Colburn_TLU=[100, 150, 1000]  Colburn_factor_TLU=[.019, .013, .002]  Re_Nu_TLU=[100, 150, 1000]  Pr_Nu_TLU=[1, 10]  Nu_TLU=[3.72, 4.21; 3.75, 4.44; 4.21, 7.15]  p0_vec=0.4 MPa  T0_vec=28 degC  mdot0=0.1 kg/s  p_nominal=0.101325 MPa  T_nominal=293.15 K
  Subsystem : Subsystem  mask{thermalR=thRes, pipeDia=pipeDiameter, pipeLen=pipeLength}
      mask prompts: thermalR "Thermal resistance (K?W)"; pipeDia "Pipe diameter (m)"; pipeLen "Pipe length (m)"
      settings: PortSchema="{\"entries\":[{\"content\":{\"sides\":[{\"content\":{\"connectorIds\":[\"LConn1\"]},\"type\":\"ConnectorPlacement.EquallySpacedRectSide\",\"uuid\":\"8372a608-b627-4dd5-95c3-37854262a040\"},{\"content\":{\"side\":\"RIGHT\"},\"type\":\"ConnectorPlacement.EquallySpacedRectSide\",\"uuid\":\"2901437e-28a5-400a-89f4-4b0cf4de73f4\"},{\"content\":{\"connectorIds\":[\"LConn2\"],\"side\":\"TOP\"},\"type\":\"ConnectorPlacement.EquallySpacedRectSide\",\"uuid\":\"68bada04-b82f-4062-ac66-e488bb531e39\"},{\"content\":{\"connectorIds\":[\"RConn1\"],\"side\":\"BOTTOM\"},\"type\":\"ConnectorPlacement.EquallySpacedRectSide\",\"uuid\":\"2ef4571e-3f54-44c8-b451-27781ea8dd24\"}]},\"type\":\"ConnectorPlacement.EquallySpacedConnector\",\"uuid\":\"734c33b2-8ec4-494c-83be-097458fcdf21\"}],\"packageUris\":[\"http://schema.mathworks.com/mf0/Connector/R2020b\"],\"version\":\"1.0\"}"
  Subsystem1 : Subsystem  mask{thermalR=thRes, pipeDia=pipeDiameter, pipeLen=pipeLength}
      mask prompts: thermalR "Thermal resistance (K?W)"; pipeDia "Pipe diameter (m)"; pipeLen "Pipe length (m)"
      settings: PortSchema="{\"entries\":[{\"content\":{\"sides\":[{\"content\":{\"connectorIds\":[\"LConn1\"]},\"type\":\"ConnectorPlacement.EquallySpacedRectSide\",\"uuid\":\"8372a608-b627-4dd5-95c3-37854262a040\"},{\"content\":{\"side\":\"RIGHT\"},\"type\":\"ConnectorPlacement.EquallySpacedRectSide\",\"uuid\":\"2901437e-28a5-400a-89f4-4b0cf4de73f4\"},{\"content\":{\"connectorIds\":[\"LConn2\"],\"side\":\"TOP\"},\"type\":\"ConnectorPlacement.EquallySpacedRectSide\",\"uuid\":\"68bada04-b82f-4062-ac66-e488bb531e39\"},{\"content\":{\"connectorIds\":[\"RConn1\"],\"side\":\"BOTTOM\"},\"type\":\"ConnectorPlacement.EquallySpacedRectSide\",\"uuid\":\"2ef4571e-3f54-44c8-b451-27781ea8dd24\"}]},\"type\":\"ConnectorPlacement.EquallySpacedConnector\",\"uuid\":\"734c33b2-8ec4-494c-83be-097458fcdf21\"}],\"packageUris\":[\"http://schema.mathworks.com/mf0/Connector/R2020b\"],\"version\":\"1.0\"}"
  Subsystem10 : Subsystem  mask{thermalR=thRes, pipeDia=pipeDiameter, pipeLen=pipeLength}
      mask prompts: thermalR "Thermal resistance (K?W)"; pipeDia "Pipe diameter (m)"; pipeLen "Pipe length (m)"
      settings: PortSchema="{\"entries\":[{\"content\":{\"sides\":[{\"content\":{\"connectorIds\":[\"LConn1\"]},\"type\":\"ConnectorPlacement.EquallySpacedRectSide\",\"uuid\":\"8372a608-b627-4dd5-95c3-37854262a040\"},{\"content\":{\"side\":\"RIGHT\"},\"type\":\"ConnectorPlacement.EquallySpacedRectSide\",\"uuid\":\"2901437e-28a5-400a-89f4-4b0cf4de73f4\"},{\"content\":{\"connectorIds\":[\"LConn2\"],\"side\":\"TOP\"},\"type\":\"ConnectorPlacement.EquallySpacedRectSide\",\"uuid\":\"68bada04-b82f-4062-ac66-e488bb531e39\"},{\"content\":{\"connectorIds\":[\"RConn1\"],\"side\":\"BOTTOM\"},\"type\":\"ConnectorPlacement.EquallySpacedRectSide\",\"uuid\":\"2ef4571e-3f54-44c8-b451-27781ea8dd24\"}]},\"type\":\"ConnectorPlacement.EquallySpacedConnector\",\"uuid\":\"734c33b2-8ec4-494c-83be-097458fcdf21\"}],\"packageUris\":[\"http://schema.mathworks.com/mf0/Connector/R2020b\"],\"version\":\"1.0\"}"
  Subsystem11 : Subsystem  mask{thermalR=thRes, pipeDia=pipeDiameter, pipeLen=pipeLength}
      mask prompts: thermalR "Thermal resistance (K?W)"; pipeDia "Pipe diameter (m)"; pipeLen "Pipe length (m)"
      settings: PortSchema="{\"entries\":[{\"content\":{\"sides\":[{\"content\":{\"connectorIds\":[\"LConn1\"]},\"type\":\"ConnectorPlacement.EquallySpacedRectSide\",\"uuid\":\"8372a608-b627-4dd5-95c3-37854262a040\"},{\"content\":{\"side\":\"RIGHT\"},\"type\":\"ConnectorPlacement.EquallySpacedRectSide\",\"uuid\":\"2901437e-28a5-400a-89f4-4b0cf4de73f4\"},{\"content\":{\"connectorIds\":[\"LConn2\"],\"side\":\"TOP\"},\"type\":\"ConnectorPlacement.EquallySpacedRectSide\",\"uuid\":\"68bada04-b82f-4062-ac66-e488bb531e39\"},{\"content\":{\"connectorIds\":[\"RConn1\"],\"side\":\"BOTTOM\"},\"type\":\"ConnectorPlacement.EquallySpacedRectSide\",\"uuid\":\"2ef4571e-3f54-44c8-b451-27781ea8dd24\"}]},\"type\":\"ConnectorPlacement.EquallySpacedConnector\",\"uuid\":\"734c33b2-8ec4-494c-83be-097458fcdf21\"}],\"packageUris\":[\"http://schema.mathworks.com/mf0/Connector/R2020b\"],\"version\":\"1.0\"}"
  Subsystem2 : Subsystem  mask{thermalR=thRes, pipeDia=pipeDiameter, pipeLen=pipeLength}
      mask prompts: thermalR "Thermal resistance (K?W)"; pipeDia "Pipe diameter (m)"; pipeLen "Pipe length (m)"
      settings: PortSchema="{\"entries\":[{\"content\":{\"sides\":[{\"content\":{\"connectorIds\":[\"LConn1\"]},\"type\":\"ConnectorPlacement.EquallySpacedRectSide\",\"uuid\":\"8372a608-b627-4dd5-95c3-37854262a040\"},{\"content\":{\"side\":\"RIGHT\"},\"type\":\"ConnectorPlacement.EquallySpacedRectSide\",\"uuid\":\"2901437e-28a5-400a-89f4-4b0cf4de73f4\"},{\"content\":{\"connectorIds\":[\"LConn2\"],\"side\":\"TOP\"},\"type\":\"ConnectorPlacement.EquallySpacedRectSide\",\"uuid\":\"68bada04-b82f-4062-ac66-e488bb531e39\"},{\"content\":{\"connectorIds\":[\"RConn1\"],\"side\":\"BOTTOM\"},\"type\":\"ConnectorPlacement.EquallySpacedRectSide\",\"uuid\":\"2ef4571e-3f54-44c8-b451-27781ea8dd24\"}]},\"type\":\"ConnectorPlacement.EquallySpacedConnector\",\"uuid\":\"734c33b2-8ec4-494c-83be-097458fcdf21\"}],\"packageUris\":[\"http://schema.mathworks.com/mf0/Connector/R2020b\"],\"version\":\"1.0\"}"
  Subsystem3 : Subsystem  mask{thermalR=thRes, pipeDia=pipeDiameter, pipeLen=pipeLength}
      mask prompts: thermalR "Thermal resistance (K?W)"; pipeDia "Pipe diameter (m)"; pipeLen "Pipe length (m)"
      settings: PortSchema="{\"entries\":[{\"content\":{\"sides\":[{\"content\":{\"connectorIds\":[\"LConn1\"]},\"type\":\"ConnectorPlacement.EquallySpacedRectSide\",\"uuid\":\"8372a608-b627-4dd5-95c3-37854262a040\"},{\"content\":{\"side\":\"RIGHT\"},\"type\":\"ConnectorPlacement.EquallySpacedRectSide\",\"uuid\":\"2901437e-28a5-400a-89f4-4b0cf4de73f4\"},{\"content\":{\"connectorIds\":[\"LConn2\"],\"side\":\"TOP\"},\"type\":\"ConnectorPlacement.EquallySpacedRectSide\",\"uuid\":\"68bada04-b82f-4062-ac66-e488bb531e39\"},{\"content\":{\"connectorIds\":[\"RConn1\"],\"side\":\"BOTTOM\"},\"type\":\"ConnectorPlacement.EquallySpacedRectSide\",\"uuid\":\"2ef4571e-3f54-44c8-b451-27781ea8dd24\"}]},\"type\":\"ConnectorPlacement.EquallySpacedConnector\",\"uuid\":\"734c33b2-8ec4-494c-83be-097458fcdf21\"}],\"packageUris\":[\"http://schema.mathworks.com/mf0/Connector/R2020b\"],\"version\":\"1.0\"}"
  Subsystem4 : Subsystem  mask{thermalR=thRes, pipeDia=pipeDiameter, pipeLen=pipeLength}
      mask prompts: thermalR "Thermal resistance (K?W)"; pipeDia "Pipe diameter (m)"; pipeLen "Pipe length (m)"
      settings: PortSchema="{\"entries\":[{\"content\":{\"sides\":[{\"content\":{\"connectorIds\":[\"LConn1\"]},\"type\":\"ConnectorPlacement.EquallySpacedRectSide\",\"uuid\":\"8372a608-b627-4dd5-95c3-37854262a040\"},{\"content\":{\"side\":\"RIGHT\"},\"type\":\"ConnectorPlacement.EquallySpacedRectSide\",\"uuid\":\"2901437e-28a5-400a-89f4-4b0cf4de73f4\"},{\"content\":{\"connectorIds\":[\"LConn2\"],\"side\":\"TOP\"},\"type\":\"ConnectorPlacement.EquallySpacedRectSide\",\"uuid\":\"68bada04-b82f-4062-ac66-e488bb531e39\"},{\"content\":{\"connectorIds\":[\"RConn1\"],\"side\":\"BOTTOM\"},\"type\":\"ConnectorPlacement.EquallySpacedRectSide\",\"uuid\":\"2ef4571e-3f54-44c8-b451-27781ea8dd24\"}]},\"type\":\"ConnectorPlacement.EquallySpacedConnector\",\"uuid\":\"734c33b2-8ec4-494c-83be-097458fcdf21\"}],\"packageUris\":[\"http://schema.mathworks.com/mf0/Connector/R2020b\"],\"version\":\"1.0\"}"
  Subsystem5 : Subsystem  mask{thermalR=thRes, pipeDia=pipeDiameter, pipeLen=pipeLength}
      mask prompts: thermalR "Thermal resistance (K?W)"; pipeDia "Pipe diameter (m)"; pipeLen "Pipe length (m)"
      settings: PortSchema="{\"entries\":[{\"content\":{\"sides\":[{\"content\":{\"connectorIds\":[\"LConn1\"]},\"type\":\"ConnectorPlacement.EquallySpacedRectSide\",\"uuid\":\"8372a608-b627-4dd5-95c3-37854262a040\"},{\"content\":{\"side\":\"RIGHT\"},\"type\":\"ConnectorPlacement.EquallySpacedRectSide\",\"uuid\":\"2901437e-28a5-400a-89f4-4b0cf4de73f4\"},{\"content\":{\"connectorIds\":[\"LConn2\"],\"side\":\"TOP\"},\"type\":\"ConnectorPlacement.EquallySpacedRectSide\",\"uuid\":\"68bada04-b82f-4062-ac66-e488bb531e39\"},{\"content\":{\"connectorIds\":[\"RConn1\"],\"side\":\"BOTTOM\"},\"type\":\"ConnectorPlacement.EquallySpacedRectSide\",\"uuid\":\"2ef4571e-3f54-44c8-b451-27781ea8dd24\"}]},\"type\":\"ConnectorPlacement.EquallySpacedConnector\",\"uuid\":\"734c33b2-8ec4-494c-83be-097458fcdf21\"}],\"packageUris\":[\"http://schema.mathworks.com/mf0/Connector/R2020b\"],\"version\":\"1.0\"}"
  Subsystem6 : Subsystem  mask{thermalR=thRes, pipeDia=pipeDiameter, pipeLen=pipeLength}
      mask prompts: thermalR "Thermal resistance (K?W)"; pipeDia "Pipe diameter (m)"; pipeLen "Pipe length (m)"
      settings: PortSchema="{\"entries\":[{\"content\":{\"sides\":[{\"content\":{\"connectorIds\":[\"LConn1\"]},\"type\":\"ConnectorPlacement.EquallySpacedRectSide\",\"uuid\":\"8372a608-b627-4dd5-95c3-37854262a040\"},{\"content\":{\"side\":\"RIGHT\"},\"type\":\"ConnectorPlacement.EquallySpacedRectSide\",\"uuid\":\"2901437e-28a5-400a-89f4-4b0cf4de73f4\"},{\"content\":{\"connectorIds\":[\"LConn2\"],\"side\":\"TOP\"},\"type\":\"ConnectorPlacement.EquallySpacedRectSide\",\"uuid\":\"68bada04-b82f-4062-ac66-e488bb531e39\"},{\"content\":{\"connectorIds\":[\"RConn1\"],\"side\":\"BOTTOM\"},\"type\":\"ConnectorPlacement.EquallySpacedRectSide\",\"uuid\":\"2ef4571e-3f54-44c8-b451-27781ea8dd24\"}]},\"type\":\"ConnectorPlacement.EquallySpacedConnector\",\"uuid\":\"734c33b2-8ec4-494c-83be-097458fcdf21\"}],\"packageUris\":[\"http://schema.mathworks.com/mf0/Connector/R2020b\"],\"version\":\"1.0\"}"
  Subsystem7 : Subsystem  mask{thermalR=thRes, pipeDia=pipeDiameter, pipeLen=pipeLength}
      mask prompts: thermalR "Thermal resistance (K?W)"; pipeDia "Pipe diameter (m)"; pipeLen "Pipe length (m)"
      settings: PortSchema="{\"entries\":[{\"content\":{\"sides\":[{\"content\":{\"connectorIds\":[\"LConn1\"]},\"type\":\"ConnectorPlacement.EquallySpacedRectSide\",\"uuid\":\"8372a608-b627-4dd5-95c3-37854262a040\"},{\"content\":{\"side\":\"RIGHT\"},\"type\":\"ConnectorPlacement.EquallySpacedRectSide\",\"uuid\":\"2901437e-28a5-400a-89f4-4b0cf4de73f4\"},{\"content\":{\"connectorIds\":[\"LConn2\"],\"side\":\"TOP\"},\"type\":\"ConnectorPlacement.EquallySpacedRectSide\",\"uuid\":\"68bada04-b82f-4062-ac66-e488bb531e39\"},{\"content\":{\"connectorIds\":[\"RConn1\"],\"side\":\"BOTTOM\"},\"type\":\"ConnectorPlacement.EquallySpacedRectSide\",\"uuid\":\"2ef4571e-3f54-44c8-b451-27781ea8dd24\"}]},\"type\":\"ConnectorPlacement.EquallySpacedConnector\",\"uuid\":\"734c33b2-8ec4-494c-83be-097458fcdf21\"}],\"packageUris\":[\"http://schema.mathworks.com/mf0/Connector/R2020b\"],\"version\":\"1.0\"}"
  Subsystem8 : Subsystem  mask{thermalR=thRes, pipeDia=pipeDiameter, pipeLen=pipeLength}
      mask prompts: thermalR "Thermal resistance (K?W)"; pipeDia "Pipe diameter (m)"; pipeLen "Pipe length (m)"
      settings: PortSchema="{\"entries\":[{\"content\":{\"sides\":[{\"content\":{\"connectorIds\":[\"LConn1\"]},\"type\":\"ConnectorPlacement.EquallySpacedRectSide\",\"uuid\":\"8372a608-b627-4dd5-95c3-37854262a040\"},{\"content\":{\"side\":\"RIGHT\"},\"type\":\"ConnectorPlacement.EquallySpacedRectSide\",\"uuid\":\"2901437e-28a5-400a-89f4-4b0cf4de73f4\"},{\"content\":{\"connectorIds\":[\"LConn2\"],\"side\":\"TOP\"},\"type\":\"ConnectorPlacement.EquallySpacedRectSide\",\"uuid\":\"68bada04-b82f-4062-ac66-e488bb531e39\"},{\"content\":{\"connectorIds\":[\"RConn1\"],\"side\":\"BOTTOM\"},\"type\":\"ConnectorPlacement.EquallySpacedRectSide\",\"uuid\":\"2ef4571e-3f54-44c8-b451-27781ea8dd24\"}]},\"type\":\"ConnectorPlacement.EquallySpacedConnector\",\"uuid\":\"734c33b2-8ec4-494c-83be-097458fcdf21\"}],\"packageUris\":[\"http://schema.mathworks.com/mf0/Connector/R2020b\"],\"version\":\"1.0\"}"
  Subsystem9 : Subsystem  mask{thermalR=thRes, pipeDia=pipeDiameter, pipeLen=pipeLength}
      mask prompts: thermalR "Thermal resistance (K?W)"; pipeDia "Pipe diameter (m)"; pipeLen "Pipe length (m)"
      settings: PortSchema="{\"entries\":[{\"content\":{\"sides\":[{\"content\":{\"connectorIds\":[\"LConn1\"]},\"type\":\"ConnectorPlacement.EquallySpacedRectSide\",\"uuid\":\"8372a608-b627-4dd5-95c3-37854262a040\"},{\"content\":{\"side\":\"RIGHT\"},\"type\":\"ConnectorPlacement.EquallySpacedRectSide\",\"uuid\":\"2901437e-28a5-400a-89f4-4b0cf4de73f4\"},{\"content\":{\"connectorIds\":[\"LConn2\"],\"side\":\"TOP\"},\"type\":\"ConnectorPlacement.EquallySpacedRectSide\",\"uuid\":\"68bada04-b82f-4062-ac66-e488bb531e39\"},{\"content\":{\"connectorIds\":[\"RConn1\"],\"side\":\"BOTTOM\"},\"type\":\"ConnectorPlacement.EquallySpacedRectSide\",\"uuid\":\"2ef4571e-3f54-44c8-b451-27781ea8dd24\"}]},\"type\":\"ConnectorPlacement.EquallySpacedConnector\",\"uuid\":\"734c33b2-8ec4-494c-83be-097458fcdf21\"}],\"packageUris\":[\"http://schema.mathworks.com/mf0/Connector/R2020b\"],\"version\":\"1.0\"}"
  H : PMIOPort  Side=Left
  B : PMIOPort  Port=2  Side=Right
  A : PMIOPort  Port=3  Side=Right
  connections:
  H/RConn1 -- Array of Thermal Nodes/RConn1
  Subsystem/LConn1 -- Array of Thermal Nodes/LConn1
  Subsystem1/LConn1 -- Array of Thermal Nodes/LConn2
  Subsystem2/LConn1 -- Array of Thermal Nodes/LConn3
  Subsystem3/LConn1 -- Array of Thermal Nodes/LConn4
  Pipe (TL)1/RConn1 -- B/RConn1
  Subsystem5/LConn2 -- Subsystem8/LConn2 -- Subsystem9/LConn2 -- Subsystem10/LConn2 -- Subsystem11/LConn2 -- Subsystem7/LConn2 -- Subsystem6/LConn2 -- Pipe (TL)1/LConn1 -- Subsystem/LConn2 -- Subsystem1/LConn2 -- Subsystem2/LConn2 -- Subsystem3/LConn2 -- Subsystem4/LConn2
  Array of Thermal Nodes/LConn5 -- Subsystem4/LConn1
  Array of Thermal Nodes/LConn6 -- Subsystem5/LConn1
  Array of Thermal Nodes/LConn8 -- Subsystem7/LConn1
  Array of Thermal Nodes/LConn7 -- Subsystem6/LConn1
  Subsystem8/LConn1 -- Array of Thermal Nodes/LConn9
  Subsystem11/LConn1 -- Array of Thermal Nodes/LConn12
  Subsystem9/LConn1 -- Array of Thermal Nodes/LConn10
  Subsystem10/LConn1 -- Array of Thermal Nodes/LConn11
  Subsystem4/RConn1 -- Subsystem7/RConn1 -- Pipe (TL)2/RConn1 -- Subsystem11/RConn1 -- Subsystem10/RConn1 -- Subsystem9/RConn1 -- Subsystem8/RConn1 -- Subsystem6/RConn1 -- Subsystem5/RConn1 -- Subsystem3/RConn1 -- Subsystem2/RConn1 -- Subsystem1/RConn1 -- Subsystem/RConn1
  A/RConn1 -- Pipe (TL)2/LConn1
  Perfect Insulator/LConn1 -- Pipe (TL)2/LConn2
  Perfect Insulator1/LConn1 -- Pipe (TL)1/LConn2

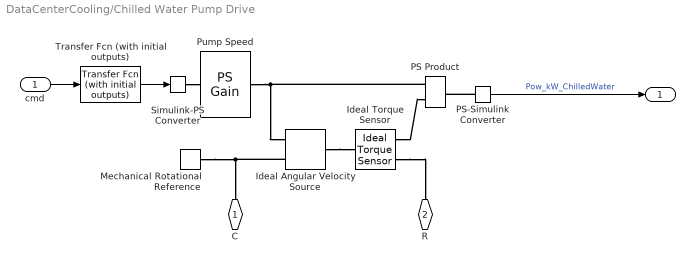
== system DataCenterCooling/Chilled Water Pump Drive ==
  cmd : Inport
  Ideal Angular Velocity Source : fl_lib/Mechanical/Mechanical Sources/Ideal Angular Velocity Source
  Ideal Torque Sensor : fl_lib/Mechanical/Mechanical Sensors/Ideal Torque Sensor
  Mechanical Rotational Reference : fl_lib/Mechanical/Rotational Elements/Mechanical Rotational Reference
  PS Product : fl_lib/Physical Signals/Functions/PS Product
  PS-Simulink Converter : nesl_utility/PS-Simulink Converter  PhysicalDomain=network_engine_domain  SubClassName=ps_output  LeftPortType=input  RightPortType=output  PseudoPeriodic=off  Frequencies=[]  VectorFormat=inherit  Unit=kW  AffineConversion=off
  Pump Speed : fl_lib/Physical Signals/Functions/PS Gain  gain=2400 rpm
  Simulink-PS Converter : nesl_utility/Simulink-PS Converter  PhysicalDomain=network_engine_domain  SubClassName=ps_input  LeftPortType=input  RightPortType=output  PseudoPeriodic=off  Frequencies=[]  NoiseDistribution=none  NoiseParameters=[]  Unit=1  AffineConversion=off  FilteringAndDerivatives=provide  SimscapeFilterOrder=1  InputFilterTimeConstant=0.001  UdotUserProvided=0
  Transfer Fcn (with initial outputs) : simulink_extras/Additional Linear/Transfer Fcn (with initial outputs)  N=[1]  D="[2  1]"  Y0=1  U0=0
  C : PMIOPort  Side=Left
  R : PMIOPort  Port=2  Side=Left
  " " : Outport
  wires:
  Transfer Fcn (with initial outputs)/1 -> Simulink-PS Converter/1
  PS-Simulink Converter/1 -> " "/1  "Pow_kW_ChilledWater"
  cmd/1 -> Transfer Fcn (with initial outputs)/1
  connections:
  Ideal Angular Velocity Source/RConn2 -- Mechanical Rotational Reference/LConn1 -- C/RConn1
  Pump Speed/RConn1 -- PS Product/LConn2 -- Ideal Angular Velocity Source/RConn1
  Simulink-PS Converter/RConn1 -- Pump Speed/LConn1
  Ideal Angular Velocity Source/LConn1 -- Ideal Torque Sensor/LConn1
  Ideal Torque Sensor/RConn1 -- R/RConn1
  Ideal Torque Sensor/RConn2 -- PS Product/LConn1
  PS-Simulink Converter/LConn1 -- PS Product/RConn1

== system DataCenterCooling/Chiller ==
  cmd : Inport
  Abstract Model : Subsystem  Tag=PublishSubsystem  VariantControl=abstract model
  Refrigeration Cycle : Subsystem  Tag=PublishSubsystem  VariantControl=refrigeration cycle
  Ae : PMIOPort  Side=Left
  Be : PMIOPort  Port=2  Side=Left
  Ac : PMIOPort  Port=3  Side=Right
  Bc : PMIOPort  Port=4  Side=Right
  Q : Outport

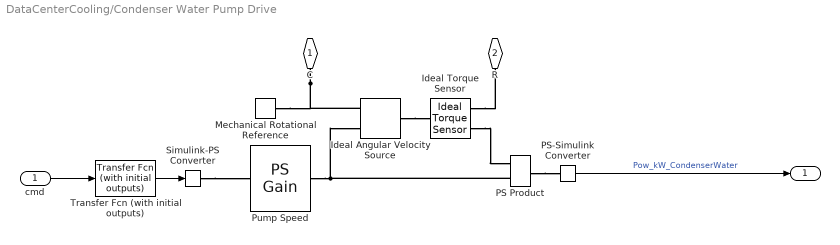
== system DataCenterCooling/Condenser Water Pump Drive ==
  cmd : Inport
  Ideal Angular Velocity Source : fl_lib/Mechanical/Mechanical Sources/Ideal Angular Velocity Source
  Ideal Torque Sensor : fl_lib/Mechanical/Mechanical Sensors/Ideal Torque Sensor
  Mechanical Rotational Reference : fl_lib/Mechanical/Rotational Elements/Mechanical Rotational Reference
  PS Product : fl_lib/Physical Signals/Functions/PS Product
  PS-Simulink Converter : nesl_utility/PS-Simulink Converter  PhysicalDomain=network_engine_domain  SubClassName=ps_output  LeftPortType=input  RightPortType=output  PseudoPeriodic=off  Frequencies=[]  VectorFormat=inherit  Unit=kW  AffineConversion=off
  Pump Speed : fl_lib/Physical Signals/Functions/PS Gain  gain=2400 rpm
  Simulink-PS Converter : nesl_utility/Simulink-PS Converter  PhysicalDomain=network_engine_domain  SubClassName=ps_input  LeftPortType=input  RightPortType=output  PseudoPeriodic=off  Frequencies=[]  NoiseDistribution=none  NoiseParameters=[]  Unit=1  AffineConversion=off  FilteringAndDerivatives=provide  SimscapeFilterOrder=1  InputFilterTimeConstant=0.001  UdotUserProvided=0
  Transfer Fcn (with initial outputs) : simulink_extras/Additional Linear/Transfer Fcn (with initial outputs)  N=[1]  D="[2  1]"  Y0=1  U0=0
  C : PMIOPort  Side=Left
  R : PMIOPort  Port=2  Side=Left
  " " : Outport
  wires:
  Transfer Fcn (with initial outputs)/1 -> Simulink-PS Converter/1
  PS-Simulink Converter/1 -> " "/1  "Pow_kW_CondenserWater"
  cmd/1 -> Transfer Fcn (with initial outputs)/1
  connections:
  C/RConn1 -- Ideal Angular Velocity Source/RConn2 -- Mechanical Rotational Reference/LConn1
  Pump Speed/RConn1 -- PS Product/LConn2 -- Ideal Angular Velocity Source/RConn1
  Simulink-PS Converter/RConn1 -- Pump Speed/LConn1
  Ideal Angular Velocity Source/LConn1 -- Ideal Torque Sensor/LConn1
  Ideal Torque Sensor/RConn1 -- R/RConn1
  Ideal Torque Sensor/RConn2 -- PS Product/LConn1
  PS Product/RConn1 -- PS-Simulink Converter/LConn1
